simulink model "lab3_madel4"  (R2022a)
settings: Solver=VariableStepAuto  StartTime=0.0  StopTime=10.0  RelTol=1e-3
libraries: slctrlblks x2
settings Model: Creator=User  LastModifiedBy=User

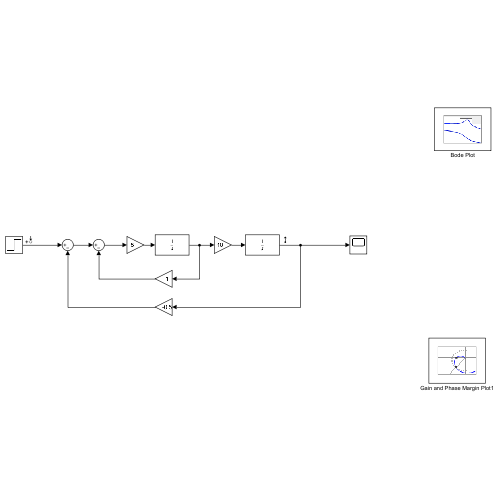
[thumbnail: Simulink's stored preview of the top-level diagram]
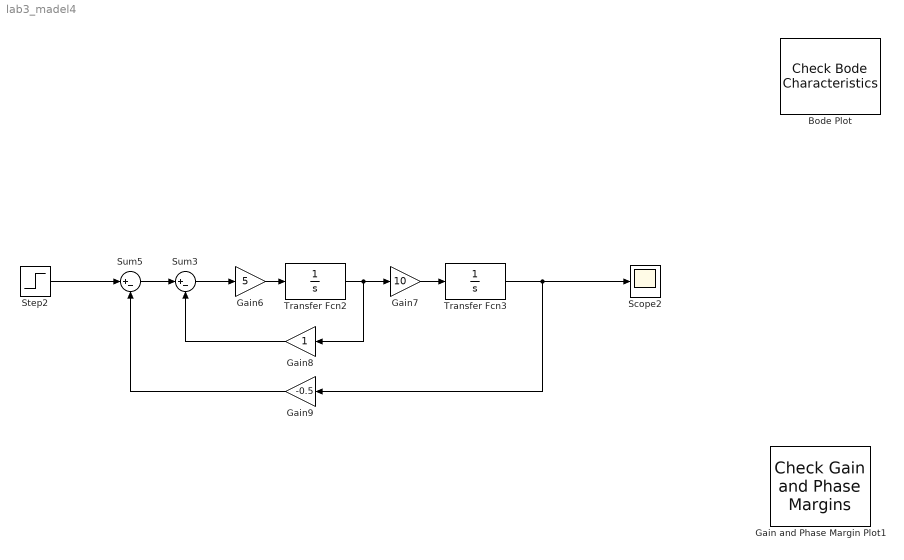
== system lab3_madel4 ==
  Bode Plot : slctrlblks/Model Verification/Check Bode  Characteristics  InstantiateOnLoad=on  SaveOperatingPoints=off  LinearizationIOs={'/Step2', 1, 'in', 'off', '';'/Transfer Fcn3', 1, 'out', 'off', ''}  LinearizeAt=SnapshotTimes  SnapshotTimes=[0]  TriggerType=rising  SampleTime=auto  RateConversionMethod=zoh  PreWarpFreq=10  UseExactDelayModel=off  UseFullBlockNameLabels=off  UseBusSignalLabels=off  enabled=on  stopWhenAssertionFail=off  export=off  ViewDlgPos=[935.4 177.8 509.6 389.6]  OpenViewOnLoad=off  LaunchViewOnOpen=on  FrequencyUnits=rad/s  MagnitudeUnits=dB  PhaseUnits=deg  TimeUnits=seconds  EnableUpperBound=off  UpperBoundFrequencies=[]  UpperBoundMagnitudes=[]  EnableLowerBound=off  LowerBoundFrequencies=[]  LowerBoundMagnitudes=[]
  Gain and Phase Margin Plot1 : slctrlblks/Model Verification/Check Gain and Phase Margins  InstantiateOnLoad=on  SaveOperatingPoints=off  LinearizationIOs={'/Step2', 1, 'in', 'off', '';'/Transfer Fcn3', 1, 'out', 'off', ''}  LinearizeAt=SnapshotTimes  SnapshotTimes=[0]  TriggerType=rising  SampleTime=auto  RateConversionMethod=zoh  PreWarpFreq=10  UseExactDelayModel=off  UseFullBlockNameLabels=off  UseBusSignalLabels=off  enabled=on  stopWhenAssertionFail=off  export=off  ViewDlgPos=[100 200 510 390]  LaunchViewOnOpen=on  OpenViewOnLoad=off  FrequencyUnits=rad/s  MagnitudeUnits=dB  PhaseUnits=deg  TimeUnits=seconds  EnableMargins=off  GainMargin=[]  PhaseMargin=[]  PlotType=nyquist  FeedbackSign=-1
      settings: SourceProductBaseCode=SD  SaveToWorkspace=off  SaveName=sys
  Gain6 : Gain  Gain=5
  Gain7 : Gain  Gain=10
  Gain8 : Gain
  Gain9 : Gain  Gain=-0.5
  Scope2 : Scope
  Step2 : Step  SampleTime=0
  Sum3 : Sum  Inputs=|+-
  Sum5 : Sum  Inputs=|+-
  Transfer Fcn2 : TransferFcn  Denominator=[1 0]
  Transfer Fcn3 : TransferFcn  Denominator=[1 0]
  wires:
  Gain9/1 -> Sum5/2
  Step2/1 -> Sum5/1
  Gain8/1 -> Sum3/2
  Sum3/1 -> Gain6/1
  Transfer Fcn2/1 -> Gain8/1, Gain7/1
  Gain6/1 -> Transfer Fcn2/1
  Gain7/1 -> Transfer Fcn3/1
  Transfer Fcn3/1 -> Gain9/1, Scope2/1
  Sum5/1 -> Sum3/1
